simulink model "concept3_simulink_RL"  (R2025a)
settings: Solver=VariableStepAuto  StartTime=0.0  StopTime=Tf  FixedStep=0.001  MaxStep=0.01  MinStep=0.0001  RelTol=1e-3
InitFcn:
  | loaded_data = load('concept3_for_sim.mat');
  | robot = loaded_data.robot;
  | robot.DataFormat = 'column';
values from neighbouring files (symbols this model uses):
  mass = 40    [RL_main.m]    (also in baseline_sim.m)
  obs_vec = opa    [RL_main.m]    (also in baseline_sim.m)
  port = data(n, :)    [RL_main.m]    (also in baseline_sim.m = port_pos_data(n,:))
  port_num = 10    [RL_main.m]    (also in baseline_sim.m)
  port_target = AB2port(port_num)    [RL_main.m]    (also in baseline_sim.m)
  q0arm = rad2deg([-1.283; -1.622; 2.2761853; -1.8021853; 1.112; 1.859; 0.05328])    [RL_main.m]    (also in baseline_sim.m)
  q0b = [1; 0; 0; 0; 0; 0; 0]    [RL_main.m]    (also in baseline_sim.m = [1;0;0;0;0;0;0])
  sat_docked = AB2port(sat_docked_num)    [RL_main.m]    (also in baseline_sim.m)
  sat_docked_num = 6    [RL_main.m]    (also in baseline_sim.m)
  sim_state = 1    [RL_main.m]    (also in baseline_sim.m)
  Tlog = 0.1    [RL_main.m]    (also in baseline_sim.m)
  use_RL = 1    [RL_main.m]    (also in baseline_sim.m)
undefined symbols (not defined in the file or in its folder): opa, target, X, Y, Z
libraries: sm_lib x133, nesl_utility x67, simulink_extras x3, rllib x2
(part 2 of 6)

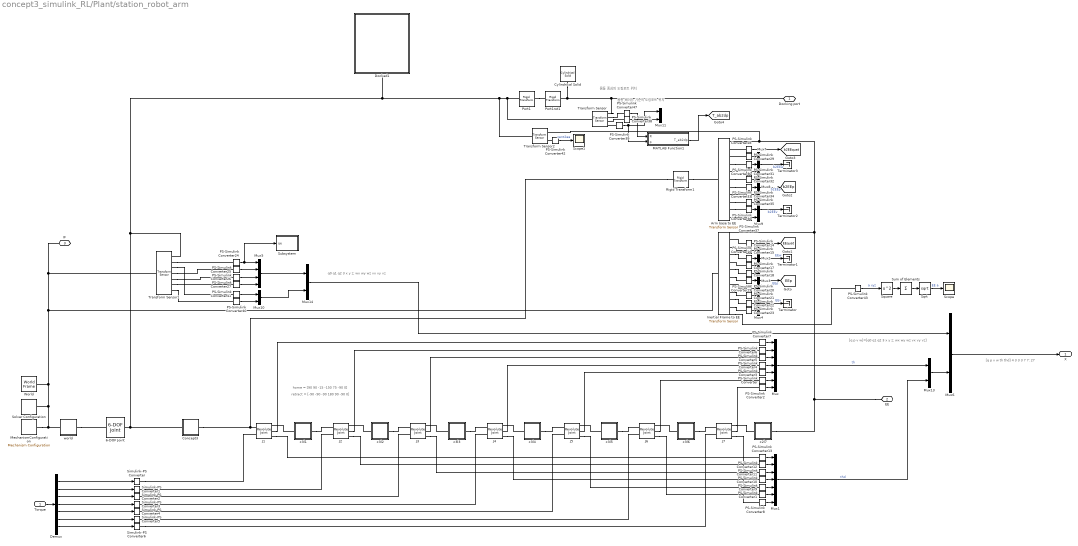
== system concept3_simulink_RL/Plant/station_robot_arm ==
  note: [q p v w th thd]
      |
      | 4 3 3 3 7 7: 27
  note: q0 q1 q2 3 x y z; wx wy wz vx vy vz
  note: 몸통 중심의 도킹포트 위치
  note: home = [90 90 -15 -150 75 -90 0]
  note: retract = [-90 -90 -90 180 90 -90 0]
  note: 몸통 베이스 기준의 도킹포트 위치
  note: [q p v w]=[q0 q1 q2 3 x y z; wx wy wz vx vy vz]
  Torque : Inport
  6-DOF Joint : sm_lib/Joints/6-DOF Joint  JointMode=Normal  CompositeWrenchDir=FollowerOnBase  CompositeWrenchFrame=BaseFrame  SenseConstraintForce=off  SenseConstraintTorque=off  SenseTotalForce=off  SenseTotalTorque=off  PxPositionTargetSpecify=on  PxPositionTargetPriority=High  PxPositionTargetValue=q0b(5)  PxPositionTargetValueUnits=m  PxVelocityTargetSpecify=off  PxVelocityTargetPriority=High  PxVelocityTargetValue=0  PxVelocityTargetValueUnits=m/s  PxEquilibriumPosition=0  PxEquilibriumPositionUnits=m  PxSpringStiffness=0  PxSpringStiffnessUnits=N/m  PxDampingCoefficient=0  PxDampingCoefficientUnits=N/(m/s)  PxLowerLimitSpecify=off  PxLowerLimitBound=-1  PxLowerLimitBoundUnits=m  PxLowerLimitStiffness=1e6  PxLowerLimitStiffnessUnits=N/m  PxLowerLimitDamping=1e3  PxLowerLimitDampingUnits=N/(m/s)  PxLowerLimitTransitionRegionWidth=1e-4  PxLowerLimitTransitionRegionWidthUnits=m  PxUpperLimitSpecify=off  PxUpperLimitBound=1  PxUpperLimitBoundUnits=m  PxUpperLimitStiffness=1e6  PxUpperLimitStiffnessUnits=N/m  PxUpperLimitDamping=1e3  PxUpperLimitDampingUnits=N/(m/s)  PxUpperLimitTransitionRegionWidth=1e-4  PxUpperLimitTransitionRegionWidthUnits=m  PxTorqueActuationMode=NoTorque  PxMotionActuationMode=ComputedMotion  PxSensePosition=off  PxSenseVelocity=off  PxSenseAcceleration=off  PxSenseTorqueForce=off  PxSenseLowerLimitTorqueForce=off  PxSenseUpperLimitTorqueForce=off  PyPositionTargetSpecify=on  PyPositionTargetPriority=High  PyPositionTargetValue=q0b(6)  PyPositionTargetValueUnits=m  PyVelocityTargetSpecify=off  PyVelocityTargetPriority=High  PyVelocityTargetValue=0  PyVelocityTargetValueUnits=m/s  PyEquilibriumPosition=0  PyEquilibriumPositionUnits=m  PySpringStiffness=0  PySpringStiffnessUnits=N/m  PyDampingCoefficient=0  PyDampingCoefficientUnits=N/(m/s)  PyLowerLimitSpecify=off  PyLowerLimitBound=-1  PyLowerLimitBoundUnits=m  PyLowerLimitStiffness=1e6  PyLowerLimitStiffnessUnits=N/m  PyLowerLimitDamping=1e3  PyLowerLimitDampingUnits=N/(m/s)  PyLowerLimitTransitionRegionWidth=1e-4  PyLowerLimitTransitionRegionWidthUnits=m  PyUpperLimitSpecify=off  PyUpperLimitBound=1  PyUpperLimitBoundUnits=m  PyUpperLimitStiffness=1e6  PyUpperLimitStiffnessUnits=N/m  PyUpperLimitDamping=1e3  PyUpperLimitDampingUnits=N/(m/s)  PyUpperLimitTransitionRegionWidth=1e-4  PyUpperLimitTransitionRegionWidthUnits=m  PyTorqueActuationMode=NoTorque  PyMotionActuationMode=ComputedMotion  PySensePosition=off  PySenseVelocity=off  PySenseAcceleration=off  PySenseTorqueForce=off  PySenseLowerLimitTorqueForce=off  PySenseUpperLimitTorqueForce=off  PzPositionTargetSpecify=on  PzPositionTargetPriority=High  PzPositionTargetValue=q0b(7)  PzPositionTargetValueUnits=m  PzVelocityTargetSpecify=off  PzVelocityTargetPriority=High  PzVelocityTargetValue=0  PzVelocityTargetValueUnits=m/s  PzEquilibriumPosition=0  PzEquilibriumPositionUnits=m  PzSpringStiffness=0  PzSpringStiffnessUnits=N/m  PzDampingCoefficient=0  PzDampingCoefficientUnits=N/(m/s)  PzLowerLimitSpecify=off  PzLowerLimitBound=-1  PzLowerLimitBoundUnits=m  PzLowerLimitStiffness=1e6  PzLowerLimitStiffnessUnits=N/m  PzLowerLimitDamping=1e3  PzLowerLimitDampingUnits=N/(m/s)  PzLowerLimitTransitionRegionWidth=1e-4  PzLowerLimitTransitionRegionWidthUnits=m  PzUpperLimitSpecify=off  PzUpperLimitBound=1  PzUpperLimitBoundUnits=m  PzUpperLimitStiffness=1e6  PzUpperLimitStiffnessUnits=N/m  PzUpperLimitDamping=1e3  PzUpperLimitDampingUnits=N/(m/s)  PzUpperLimitTransitionRegionWidth=1e-4  PzUpperLimitTransitionRegionWidthUnits=m  PzTorqueActuationMode=NoTorque  PzMotionActuationMode=ComputedMotion  PzSensePosition=off  PzSenseVelocity=off  PzSenseAcceleration=off  PzSenseTorqueForce=off  PzSenseLowerLimitTorqueForce=off  PzSenseUpperLimitTorqueForce=off  SphPositionTargetSpecify=on  SphPositionTargetPriority=High  SphPositionTargetRotationMethod=Quaternion  SphPositionTargetFollAlignAxisA=+X  SphPositionTargetBaseAlignAxisA=+Y  SphPositionTargetFollAlignAxisB=+Y  SphPositionTargetBaseAlignAxisB=+Z  SphPositionTargetRotationStandardAxis=+Y  SphPositionTargetRotationAngle=0  SphPositionTargetRotationAngleUnits=deg  SphPositionTargetRotationArbitraryAxis=[0 0 1]  SphPositionTargetRotationSequenceAxes=FollowerAxes  SphPositionTargetRotationSequence=XYX  SphPositionTargetRotationSequenceAngles=[0 0 0]  SphPositionTargetRotationSequenceAnglesUnits=deg  SphPositionTargetRotationMatrix=[1 0 0;0 1 0;0 0 1]  SphPositionTargetQuaternion=q0b(1:4)  SphVelocityTargetSpecify=off  SphVelocityTargetPriority=High  SphVelocityTargetValue=[0 0 0]  SphVelocityTargetValueUnits=deg/s  SphVelocityTargetInFollowerFrame=on  SphEqPosRotationMethod=None  SphEqPosFollAlignAxisA=+X  SphEqPosBaseAlignAxisA=+Y  SphEqPosFollAlignAxisB=+Y  SphEqPosBaseAlignAxisB=+Z  SphEqPosRotationStandardAxis=+Z  SphEqPosRotationAngle=0  SphEqPosRotationAngleUnits=deg  SphEqPosRotationArbitraryAxis=[0 0 1]  SphEqPosRotationSequenceAxes=FollowerAxes  SphEqPosRotationSequence=XYX  SphEqPosRotationSequenceAngles=[0 0 0]  SphEqPosRotationSequenceAnglesUnits=deg  SphEqPosRotationMatrix=[1 0 0;0 1 0;0 0 1]  SphEqPosQuaternion=[1 0 0 0]  SphSpringStiffness=0  SphSpringStiffnessUnits=N*m/deg  SphDampingCoefficient=0  SphDampingCoefficientUnits=N*m/(deg/s)  SphLowerLimitSpecify=off  SphLowerLimitBound=15  SphLowerLimitBoundUnits=deg  SphLowerLimitStiffness=1e4  SphLowerLimitStiffnessUnits=N*m/deg  SphLowerLimitDamping=10  SphLowerLimitDampingUnits=N*m/(deg/s)  SphLowerLimitTransitionRegionWidth=0.1  SphLowerLimitTransitionRegionWidthUnits=deg  SphUpperLimitSpecify=off  SphUpperLimitBound=45  SphUpperLimitBoundUnits=deg  SphUpperLimitStiffness=1e4  SphUpperLimitStiffnessUnits=N*m/deg  SphUpperLimitDamping=10  SphUpperLimitDampingUnits=N*m/(deg/s)  SphUpperLimitTransitionRegionWidth=0.1  SphUpperLimitTransitionRegionWidthUnits=deg  SphTorqueActuationMode=InputTorque  SphActuateTorqueX=off  SphActuateTorqueY=off  SphActuateTorqueZ=off  SphActuateTorque=off  SphActuationFrame=BaseFrame  SphSensePosition=off  SphSenseVelocityX=off  SphSenseVelocityY=off  SphSenseVelocityZ=off  SphSenseVelocity=off  SphSenseAccelerationX=off  SphSenseAccelerationY=off  SphSenseAccelerationZ=off  SphSenseAcceleration=off  SphSenseLowerLimitTorqueMag=off  SphSenseUpperLimitTorqueMag=off  SphSensingFrame=BaseFrame
  Arm base to EE : sm_lib/Frames and Transforms/Transform Sensor  MeasurementFrame=Base  RotationSequence=XYX  SenseAngle=off  SenseAxis=off  SenseQ=on  SenseR=off  SenseRotationSequence=off  SenseOmegaX=on  SenseOmegaY=on  SenseOmegaZ=on  SenseOmega=off  SenseQDot=off  SenseRDot=off  SenseRotationSequenceDot=off  SenseAlphaX=off  SenseAlphaY=off  SenseAlphaZ=off  SenseAlpha=off  SenseQDDot=off  SenseRDDot=off  SenseX=on  SenseY=on  SenseZ=on  SenseXYZ=off  SenseRad=off  SenseAzim=off  SenseDist=off  SenseInc=off  SenseXDot=on  SenseYDot=on  SenseZDot=on  SenseXYZDot=off  SenseRadDot=off  SenseAzimDot=off  SenseDistDot=off  SenseIncDot=off  SenseXDDot=off  SenseYDDot=off  SenseZDDot=off  SenseXYZDDot=off  SenseRadDDot=off  SenseAzimDDot=off  SenseDistDDot=off  SenseIncDDot=off
  Concept3 : Subsystem
  Cylindrical Solid : sm_lib/Body Elements/Cylindrical Solid  CylinderRadius=0.05  CylinderRadiusUnits=m  CylinderLength=0.01  CylinderLengthUnits=m  ExportEntireGeometry=off  InertiaType=CalculateFromGeometry  BasedOnType=Mass  Density=1000  DensityUnits=kg/m^3  Mass=0  MassUnits=kg  CenterOfMass=[0 0 0]  CenterOfMassUnits=m  MomentsOfInertia=[1 1 1]  MomentsOfInertiaUnits=kg*m^2  ProductsOfInertia=[0 0 0]  ProductsOfInertiaUnits=kg*m^2  GraphicType=FromGeometry  MarkerShape=Sphere  MarkerSize=10  GraphicVisPropType=SimpleVisualProperties  GraphicDiffuseColor=[0 1 1]  GraphicOpacity=0.5  GraphicSpecularColor=[0.5 0.5 0.5 1]  GraphicAmbientColor=[0.15 0.15 0.15 1]  GraphicEmissiveColor=[0.0 0.0 0.0 1.0]  GraphicShininess=100  DoExposeReferenceFrame=on  SerializedFrames=<Frames/>
  Demux : Demux  Outputs=7
  Docked1 : Subsystem
  Inertial Frame to EE : sm_lib/Frames and Transforms/Transform Sensor  MeasurementFrame=World  RotationSequence=XYX  SenseAngle=off  SenseAxis=off  SenseQ=on  SenseR=off  SenseRotationSequence=off  SenseOmegaX=on  SenseOmegaY=on  SenseOmegaZ=on  SenseOmega=off  SenseQDot=off  SenseRDot=off  SenseRotationSequenceDot=off  SenseAlphaX=off  SenseAlphaY=off  SenseAlphaZ=off  SenseAlpha=off  SenseQDDot=off  SenseRDDot=off  SenseX=on  SenseY=on  SenseZ=on  SenseXYZ=off  SenseRad=off  SenseAzim=off  SenseDist=off  SenseInc=off  SenseXDot=on  SenseYDot=on  SenseZDot=on  SenseXYZDot=off  SenseRadDot=off  SenseAzimDot=off  SenseDistDot=off  SenseIncDot=off  SenseXDDot=off  SenseYDDot=off  SenseZDDot=off  SenseXYZDDot=on  SenseRadDDot=off  SenseAzimDDot=off  SenseDistDDot=off  SenseIncDDot=off
  J1 : sm_lib/Joints/Revolute Joint  JointMode=Normal  CompositeWrenchDir=FollowerOnBase  CompositeWrenchFrame=BaseFrame  SenseConstraintForce=off  SenseConstraintTorque=off  SenseTotalForce=off  SenseTotalTorque=off  PositionTargetSpecify=on  PositionTargetPriority=High  PositionTargetValue=q0arm(1)  PositionTargetValueUnits=deg  VelocityTargetSpecify=off  VelocityTargetPriority=High  VelocityTargetValue=0  VelocityTargetValueUnits=deg/s  EquilibriumPosition=0  EquilibriumPositionUnits=deg  SpringStiffness=0  SpringStiffnessUnits=N*m/deg  DampingCoefficient=0  DampingCoefficientUnits=kg*m^2/(rad*s)  LowerLimitSpecify=off  LowerLimitBound=-90  LowerLimitBoundUnits=deg  LowerLimitStiffness=1e4  LowerLimitStiffnessUnits=N*m/deg  LowerLimitDamping=10  LowerLimitDampingUnits=N*m/(deg/s)  LowerLimitTransitionRegionWidth=0.1  LowerLimitTransitionRegionWidthUnits=deg  UpperLimitSpecify=off  UpperLimitBound=90  UpperLimitBoundUnits=deg  UpperLimitStiffness=1e4  UpperLimitStiffnessUnits=N*m/deg  UpperLimitDamping=10  UpperLimitDampingUnits=N*m/(deg/s)  UpperLimitTransitionRegionWidth=0.1  UpperLimitTransitionRegionWidthUnits=deg  TorqueActuationMode=InputTorque  MotionActuationMode=ComputedMotion  SensePosition=on  SenseVelocity=on  SenseAcceleration=off  SenseTorqueForce=off  SenseLowerLimitTorqueForce=off  SenseUpperLimitTorqueForce=off
  J2 : sm_lib/Joints/Revolute Joint  JointMode=Normal  CompositeWrenchDir=FollowerOnBase  CompositeWrenchFrame=BaseFrame  SenseConstraintForce=off  SenseConstraintTorque=off  SenseTotalForce=off  SenseTotalTorque=off  PositionTargetSpecify=on  PositionTargetPriority=High  PositionTargetValue=q0arm(2)  PositionTargetValueUnits=deg  VelocityTargetSpecify=off  VelocityTargetPriority=High  VelocityTargetValue=0  VelocityTargetValueUnits=deg/s  EquilibriumPosition=0  EquilibriumPositionUnits=deg  SpringStiffness=0  SpringStiffnessUnits=N*m/deg  DampingCoefficient=0  DampingCoefficientUnits=kg*m^2/(rad*s)  LowerLimitSpecify=off  LowerLimitBound=-90  LowerLimitBoundUnits=deg  LowerLimitStiffness=1e4  LowerLimitStiffnessUnits=N*m/deg  LowerLimitDamping=10  LowerLimitDampingUnits=N*m/(deg/s)  LowerLimitTransitionRegionWidth=0.1  LowerLimitTransitionRegionWidthUnits=deg  UpperLimitSpecify=off  UpperLimitBound=90  UpperLimitBoundUnits=deg  UpperLimitStiffness=1e4  UpperLimitStiffnessUnits=N*m/deg  UpperLimitDamping=10  UpperLimitDampingUnits=N*m/(deg/s)  UpperLimitTransitionRegionWidth=0.1  UpperLimitTransitionRegionWidthUnits=deg  TorqueActuationMode=InputTorque  MotionActuationMode=ComputedMotion  SensePosition=on  SenseVelocity=on  SenseAcceleration=off  SenseTorqueForce=off  SenseLowerLimitTorqueForce=off  SenseUpperLimitTorqueForce=off
  J3 : sm_lib/Joints/Revolute Joint  JointMode=Normal  CompositeWrenchDir=FollowerOnBase  CompositeWrenchFrame=BaseFrame  SenseConstraintForce=off  SenseConstraintTorque=off  SenseTotalForce=off  SenseTotalTorque=off  PositionTargetSpecify=on  PositionTargetPriority=High  PositionTargetValue=q0arm(3)  PositionTargetValueUnits=deg  VelocityTargetSpecify=off  VelocityTargetPriority=High  VelocityTargetValue=0  VelocityTargetValueUnits=deg/s  EquilibriumPosition=0  EquilibriumPositionUnits=deg  SpringStiffness=0  SpringStiffnessUnits=N*m/deg  DampingCoefficient=0  DampingCoefficientUnits=kg*m^2/(rad*s)  LowerLimitSpecify=off  LowerLimitBound=-90  LowerLimitBoundUnits=deg  LowerLimitStiffness=1e4  LowerLimitStiffnessUnits=N*m/deg  LowerLimitDamping=10  LowerLimitDampingUnits=N*m/(deg/s)  LowerLimitTransitionRegionWidth=0.1  LowerLimitTransitionRegionWidthUnits=deg  UpperLimitSpecify=off  UpperLimitBound=90  UpperLimitBoundUnits=deg  UpperLimitStiffness=1e4  UpperLimitStiffnessUnits=N*m/deg  UpperLimitDamping=10  UpperLimitDampingUnits=N*m/(deg/s)  UpperLimitTransitionRegionWidth=0.1  UpperLimitTransitionRegionWidthUnits=deg  TorqueActuationMode=InputTorque  MotionActuationMode=ComputedMotion  SensePosition=on  SenseVelocity=on  SenseAcceleration=off  SenseTorqueForce=off  SenseLowerLimitTorqueForce=off  SenseUpperLimitTorqueForce=off
  J4 : sm_lib/Joints/Revolute Joint  JointMode=Normal  CompositeWrenchDir=FollowerOnBase  CompositeWrenchFrame=BaseFrame  SenseConstraintForce=off  SenseConstraintTorque=off  SenseTotalForce=off  SenseTotalTorque=off  PositionTargetSpecify=on  PositionTargetPriority=High  PositionTargetValue=q0arm(4)  PositionTargetValueUnits=deg  VelocityTargetSpecify=off  VelocityTargetPriority=High  VelocityTargetValue=0  VelocityTargetValueUnits=deg/s  EquilibriumPosition=0  EquilibriumPositionUnits=deg  SpringStiffness=0  SpringStiffnessUnits=N*m/deg  DampingCoefficient=0  DampingCoefficientUnits=kg*m^2/(rad*s)  LowerLimitSpecify=off  LowerLimitBound=-90  LowerLimitBoundUnits=deg  LowerLimitStiffness=1e4  LowerLimitStiffnessUnits=N*m/deg  LowerLimitDamping=10  LowerLimitDampingUnits=N*m/(deg/s)  LowerLimitTransitionRegionWidth=0.1  LowerLimitTransitionRegionWidthUnits=deg  UpperLimitSpecify=off  UpperLimitBound=90  UpperLimitBoundUnits=deg  UpperLimitStiffness=1e4  UpperLimitStiffnessUnits=N*m/deg  UpperLimitDamping=10  UpperLimitDampingUnits=N*m/(deg/s)  UpperLimitTransitionRegionWidth=0.1  UpperLimitTransitionRegionWidthUnits=deg  TorqueActuationMode=InputTorque  MotionActuationMode=ComputedMotion  SensePosition=on  SenseVelocity=on  SenseAcceleration=off  SenseTorqueForce=off  SenseLowerLimitTorqueForce=off  SenseUpperLimitTorqueForce=off
  J5 : sm_lib/Joints/Revolute Joint  JointMode=Normal  CompositeWrenchDir=FollowerOnBase  CompositeWrenchFrame=BaseFrame  SenseConstraintForce=off  SenseConstraintTorque=off  SenseTotalForce=off  SenseTotalTorque=off  PositionTargetSpecify=on  PositionTargetPriority=High  PositionTargetValue=q0arm(5)  PositionTargetValueUnits=deg  VelocityTargetSpecify=off  VelocityTargetPriority=High  VelocityTargetValue=0  VelocityTargetValueUnits=deg/s  EquilibriumPosition=0  EquilibriumPositionUnits=deg  SpringStiffness=0  SpringStiffnessUnits=N*m/deg  DampingCoefficient=0  DampingCoefficientUnits=kg*m^2/(rad*s)  LowerLimitSpecify=off  LowerLimitBound=-90  LowerLimitBoundUnits=deg  LowerLimitStiffness=1e4  LowerLimitStiffnessUnits=N*m/deg  LowerLimitDamping=10  LowerLimitDampingUnits=N*m/(deg/s)  LowerLimitTransitionRegionWidth=0.1  LowerLimitTransitionRegionWidthUnits=deg  UpperLimitSpecify=off  UpperLimitBound=90  UpperLimitBoundUnits=deg  UpperLimitStiffness=1e4  UpperLimitStiffnessUnits=N*m/deg  UpperLimitDamping=10  UpperLimitDampingUnits=N*m/(deg/s)  UpperLimitTransitionRegionWidth=0.1  UpperLimitTransitionRegionWidthUnits=deg  TorqueActuationMode=InputTorque  MotionActuationMode=ComputedMotion  SensePosition=on  SenseVelocity=on  SenseAcceleration=off  SenseTorqueForce=off  SenseLowerLimitTorqueForce=off  SenseUpperLimitTorqueForce=off
  J6 : sm_lib/Joints/Revolute Joint  JointMode=Normal  CompositeWrenchDir=FollowerOnBase  CompositeWrenchFrame=BaseFrame  SenseConstraintForce=off  SenseConstraintTorque=off  SenseTotalForce=off  SenseTotalTorque=off  PositionTargetSpecify=on  PositionTargetPriority=High  PositionTargetValue=q0arm(6)  PositionTargetValueUnits=deg  VelocityTargetSpecify=off  VelocityTargetPriority=High  VelocityTargetValue=0  VelocityTargetValueUnits=deg/s  EquilibriumPosition=0  EquilibriumPositionUnits=deg  SpringStiffness=0  SpringStiffnessUnits=N*m/deg  DampingCoefficient=0  DampingCoefficientUnits=kg*m^2/(rad*s)  LowerLimitSpecify=off  LowerLimitBound=-90  LowerLimitBoundUnits=deg  LowerLimitStiffness=1e4  LowerLimitStiffnessUnits=N*m/deg  LowerLimitDamping=10  LowerLimitDampingUnits=N*m/(deg/s)  LowerLimitTransitionRegionWidth=0.1  LowerLimitTransitionRegionWidthUnits=deg  UpperLimitSpecify=off  UpperLimitBound=90  UpperLimitBoundUnits=deg  UpperLimitStiffness=1e4  UpperLimitStiffnessUnits=N*m/deg  UpperLimitDamping=10  UpperLimitDampingUnits=N*m/(deg/s)  UpperLimitTransitionRegionWidth=0.1  UpperLimitTransitionRegionWidthUnits=deg  TorqueActuationMode=InputTorque  MotionActuationMode=ComputedMotion  SensePosition=on  SenseVelocity=on  SenseAcceleration=off  SenseTorqueForce=off  SenseLowerLimitTorqueForce=off  SenseUpperLimitTorqueForce=off
  J7 : sm_lib/Joints/Revolute Joint  JointMode=Normal  CompositeWrenchDir=FollowerOnBase  CompositeWrenchFrame=BaseFrame  SenseConstraintForce=off  SenseConstraintTorque=off  SenseTotalForce=off  SenseTotalTorque=off  PositionTargetSpecify=on  PositionTargetPriority=High  PositionTargetValue=q0arm(7)  PositionTargetValueUnits=deg  VelocityTargetSpecify=off  VelocityTargetPriority=High  VelocityTargetValue=0  VelocityTargetValueUnits=deg/s  EquilibriumPosition=0  EquilibriumPositionUnits=deg  SpringStiffness=0  SpringStiffnessUnits=N*m/deg  DampingCoefficient=0  DampingCoefficientUnits=kg*m^2/(rad*s)  LowerLimitSpecify=off  LowerLimitBound=-90  LowerLimitBoundUnits=deg  LowerLimitStiffness=1e4  LowerLimitStiffnessUnits=N*m/deg  LowerLimitDamping=10  LowerLimitDampingUnits=N*m/(deg/s)  LowerLimitTransitionRegionWidth=0.1  LowerLimitTransitionRegionWidthUnits=deg  UpperLimitSpecify=off  UpperLimitBound=90  UpperLimitBoundUnits=deg  UpperLimitStiffness=1e4  UpperLimitStiffnessUnits=N*m/deg  UpperLimitDamping=10  UpperLimitDampingUnits=N*m/(deg/s)  UpperLimitTransitionRegionWidth=0.1  UpperLimitTransitionRegionWidthUnits=deg  TorqueActuationMode=InputTorque  MotionActuationMode=ComputedMotion  SensePosition=on  SenseVelocity=on  SenseAcceleration=off  SenseTorqueForce=off  SenseLowerLimitTorqueForce=off  SenseUpperLimitTorqueForce=off
  MATLAB Function1 : MATLAB Function  TreatAsAtomicUnit=on
  MechanismConfiguration : sm_lib/Utilities/Mechanism Configuration  UniformGravity=Constant  GravityVector=[0, 0, 0]  GravityVectorUnits=m/s^2  LinearizationDelta=0.001  JointModeTransitionNonlinearIterations=2
  Mux : Mux  Inputs=7
  Mux1 : Mux  Inputs=7
  Mux{6,10..11,13..14} (5 alike) : Mux  Inputs=2
  Mux{2..4,7..9} (6 alike) : Mux  Inputs=3
  Mux5 : Mux
  PS-Simulink Converter{,1..43,47} (45 alike) : nesl_utility/PS-Simulink Converter  PhysicalDomain=network_engine_domain  SubClassName=ps_output  LeftPortType=input  RightPortType=output  PseudoPeriodic=off  Frequencies=[]  VectorFormat=inherit  Unit=inherit  AffineConversion=off
  Port1 : sm_lib/Frames and Transforms/Rigid Transform  RotationMethod=None  FollAlignAxisA=+X  BaseAlignAxisA=+Y  FollAlignAxisB=+Y  BaseAlignAxisB=+Z  RotationStandardAxis=+Z  RotationAngle=0  RotationAngleUnits=deg  RotationArbitraryAxis=[0 0 1]  RotationSequenceAxes=FollowerAxes  RotationSequence=XYX  RotationSequenceAngles=[0 0 0]  RotationSequenceAnglesUnits=deg  RotationMatrix=[1 0 0;0 1 0;0 0 1]  Quaternion=[1 0 0 0]  TranslationMethod=Cartesian  TranslationCartesianOffset=port_target(1:3)  TranslationCartesianOffsetUnits=m  TranslationStandardAxis=+Z  TranslationStandardOffset=0  TranslationStandardOffsetUnits=m  TranslationROffset=0  TranslationROffsetUnits=m  TranslationThetaOffset=0  TranslationThetaOffsetUnits=deg  TranslationZOffset=0  TranslationZOffsetUnits=m
  Port1rot1 : sm_lib/Frames and Transforms/Rigid Transform  RotationMethod=RotationSequence  FollAlignAxisA=+X  BaseAlignAxisA=+Y  FollAlignAxisB=+Y  BaseAlignAxisB=+Z  RotationStandardAxis=+Z  RotationAngle=0  RotationAngleUnits=deg  RotationArbitraryAxis=[0 0 1]  RotationSequenceAxes=FollowerAxes  RotationSequence=ZYX  RotationSequenceAngles=port_target(4:6)  RotationSequenceAnglesUnits=deg  RotationMatrix=[1 0 0;0 1 0;0 0 1]  Quaternion=[1 0 0 0]  TranslationMethod=None  TranslationCartesianOffset=[0.9 -0.25 -0.05]  TranslationCartesianOffsetUnits=m  TranslationStandardAxis=+Z  TranslationStandardOffset=0  TranslationStandardOffsetUnits=m  TranslationROffset=0  TranslationROffsetUnits=m  TranslationThetaOffset=0  TranslationThetaOffsetUnits=deg  TranslationZOffset=0  TranslationZOffsetUnits=m
  Rigid Transform1 : sm_lib/Frames and Transforms/Rigid Transform  RotationMethod=StandardAxis  FollAlignAxisA=+X  BaseAlignAxisA=+Y  FollAlignAxisB=+Y  BaseAlignAxisB=+Z  RotationStandardAxis=+Z  RotationAngle=0  RotationAngleUnits=deg  RotationArbitraryAxis=[0 0 1]  RotationSequenceAxes=FollowerAxes  RotationSequence=XYX  RotationSequenceAngles=[0 0 0]  RotationSequenceAnglesUnits=deg  RotationMatrix=[1 0 0;0 1 0;0 0 1]  Quaternion=[1 0 0 0]  TranslationMethod=None  TranslationCartesianOffset=[0 0 0]  TranslationCartesianOffsetUnits=m  TranslationStandardAxis=+Z  TranslationStandardOffset=0  TranslationStandardOffsetUnits=m  TranslationROffset=0  TranslationROffsetUnits=m  TranslationThetaOffset=0  TranslationThetaOffsetUnits=deg  TranslationZOffset=0  TranslationZOffsetUnits=m
  Scope : Scope
  Scope1 : Scope
      settings: DataLoggingVariableName=ScopeData3
  Simulink-PS Converter{,1..6} (7 alike) : nesl_utility/Simulink-PS Converter  PhysicalDomain=network_engine_domain  SubClassName=ps_input  LeftPortType=input  RightPortType=output  PseudoPeriodic=off  Frequencies=[]  NoiseDistribution=none  NoiseParameters=[]  Unit=1  AffineConversion=off  FilteringAndDerivatives=provide  SimscapeFilterOrder=1  InputFilterTimeConstant=0.001  UdotUserProvided=0
  Solver Configuration : nesl_utility/Solver Configuration  PhysicalDomain=network_engine_domain  SubClassName=solver  LeftPortType=input  RightPortType=generic  Tones=[]  Harmonics=[]  SimulateNoise=off  Profile=off  UseLocalSampling=off  EnableSwitchedLinearOptims=on  FrequencyDomain=off  UseCCode=off  RelTol=0.001  AbsTol=0.001  MinStep=1e-09  ToWorkspace=off  RevertToSquareIcSolve=off  NumHomotopyIterations=100  PhasorMode=off  PhasorModeNumHarmonics=1  ConsistencySolver=NEWTON_XTOL_AFTER_FTOL  IndexReductionMethod=DerivativeReplacement  DoDC=off  ResidualTolerance=1e-09  ConsistencyTolSource=GLOBAL  ConsistencyAbsTol=0.001  ConsistencyRelTol=0.001  ConsistencyTolFactor=0.001  UseLocalSolver=off  LocalSolverChoice=NE_BACKWARD_EULER_ADVANCER  ResolveIndetEquations=on  FunctionEvalNumThread=1  LocalSolverSampleTime=0.001  DoFixedCost=off  MaxNonlinIter=3  MaxModeIter=2  ComputeImpulses=off  ImpulseIterations=2  LinearAlgebra=auto  LinearAlgebraNumThread=0  EquationFormulation=NE_TIME_EF  DelaysMemoryBudget=1024  AutomaticFiltering=on  FilteringTimeConstant=0.001  PartitionStorageMethod=AS_NEEDED  PartitionMemoryBudget=1024  PartitionMethod=ROBUST  MultibodyUseLocalSolver=off  MultibodyLocalSolverChoice=ODE1  MultibodyLocalSolverSampleTime=0.001
  Sqrt : Sqrt
  Square : Math  Operator=square
  Subsystem : Subsystem
  Sum of Elements : Sum  Inputs=+
  Terminator{,1..3} (4 alike) : Terminator
  Transform Sensor : sm_lib/Frames and Transforms/Transform Sensor  MeasurementFrame=Base  RotationSequence=ZYX  SenseAngle=off  SenseAxis=off  SenseQ=off  SenseR=on  SenseRotationSequence=on  SenseOmegaX=off  SenseOmegaY=off  SenseOmegaZ=off  SenseOmega=off  SenseQDot=off  SenseRDot=off  SenseRotationSequenceDot=off  SenseAlphaX=off  SenseAlphaY=off  SenseAlphaZ=off  SenseAlpha=off  SenseQDDot=off  SenseRDDot=off  SenseX=off  SenseY=off  SenseZ=off  SenseXYZ=on  SenseRad=off  SenseAzim=off  SenseDist=off  SenseInc=off  SenseXDot=off  SenseYDot=off  SenseZDot=off  SenseXYZDot=off  SenseRadDot=off  SenseAzimDot=off  SenseDistDot=off  SenseIncDot=off  SenseXDDot=off  SenseYDDot=off  SenseZDDot=off  SenseXYZDDot=off  SenseRadDDot=off  SenseAzimDDot=off  SenseDistDDot=off  SenseIncDDot=off
  Transform Sensor1 : sm_lib/Frames and Transforms/Transform Sensor  MeasurementFrame=World  RotationSequence=XYX  SenseAngle=off  SenseAxis=off  SenseQ=on  SenseR=off  SenseRotationSequence=off  SenseOmegaX=off  SenseOmegaY=off  SenseOmegaZ=off  SenseOmega=on  SenseQDot=off  SenseRDot=off  SenseRotationSequenceDot=off  SenseAlphaX=off  SenseAlphaY=off  SenseAlphaZ=off  SenseAlpha=off  SenseQDDot=off  SenseRDDot=off  SenseX=on  SenseY=on  SenseZ=on  SenseXYZ=off  SenseRad=off  SenseAzim=off  SenseDist=off  SenseInc=off  SenseXDot=off  SenseYDot=off  SenseZDot=off  SenseXYZDot=on  SenseRadDot=off  SenseAzimDot=off  SenseDistDot=off  SenseIncDot=off  SenseXDDot=off  SenseYDDot=off  SenseZDDot=off  SenseXYZDDot=off  SenseRadDDot=off  SenseAzimDDot=off  SenseDistDDot=off  SenseIncDDot=off
  Transform Sensor2 : sm_lib/Frames and Transforms/Transform Sensor  MeasurementFrame=Base  RotationSequence=ZYX  SenseAngle=off  SenseAxis=off  SenseQ=off  SenseR=off  SenseRotationSequence=off  SenseOmegaX=off  SenseOmegaY=off  SenseOmegaZ=off  SenseOmega=off  SenseQDot=off  SenseRDot=off  SenseRotationSequenceDot=off  SenseAlphaX=off  SenseAlphaY=off  SenseAlphaZ=off  SenseAlpha=off  SenseQDDot=off  SenseRDDot=off  SenseX=off  SenseY=off  SenseZ=off  SenseXYZ=on  SenseRad=off  SenseAzim=off  SenseDist=off  SenseInc=off  SenseXDot=off  SenseYDot=off  SenseZDot=off  SenseXYZDot=off  SenseRadDot=off  SenseAzimDot=off  SenseDistDot=off  SenseIncDot=off  SenseXDDot=off  SenseYDDot=off  SenseZDDot=off  SenseXYZDDot=off  SenseRadDDot=off  SenseAzimDDot=off  SenseDistDDot=off  SenseIncDDot=off
  World : sm_lib/Frames and Transforms/World Frame
  c2l7 : Subsystem
  c3l1 : Subsystem
  c3l2 : Subsystem
  c3l3 : Subsystem
  c3l4 : Subsystem
  c3l5 : Subsystem
  c3l6 : Subsystem
  world : Subsystem
  Docking port : PMIOPort  Side=Right
  EE : PMIOPort  Port=2  Side=Right
  IF : PMIOPort  Port=3  Side=Right
  X : Outport
  tag scope: EEp=global, EEquat=global, T_ab2dp=global, b2EEp=global, b2EEquat=global
  wires:
  PS-Simulink Converter4/1 -> Mux/4
  Mux4/1 -> Terminator/1  "EEv"
  Demux/5 -> Simulink-PS Converter4/1
  PS-Simulink Converter9/1 -> Mux1/5
  PS-Simulink Converter15/1 -> Mux2/1
  Torque/1 -> Demux/1
  PS-Simulink Converter26/1 -> Mux5/3
  PS-Simulink Converter13/1 -> Mux1/1
  PS-Simulink Converter8/1 -> Mux1/7
  Mux2/1 -> Terminator1/1  "EEw"
  PS-Simulink Converter23/1 -> Mux4/3
  PS-Simulink Converter11/1 -> Mux1/3
  PS-Simulink Converter5/1 -> Mux/3
  Demux/4 -> Simulink-PS Converter3/1
  PS-Simulink Converter1/1 -> Mux1/6
  Demux/2 -> Simulink-PS Converter1/1
  PS-Simulink Converter22/1 -> Mux4/2
  PS-Simulink Converter21/1 -> Mux4/1
  Demux/3 -> Simulink-PS Converter2/1
  PS-Simulink Converter19/1 -> Mux3/2
  PS-Simulink Converter6/1 -> Mux/2
  PS-Simulink Converter20/1 -> Mux3/3
  PS-Simulink Converter3/1 -> Mux/5
  PS-Simulink Converter17/1 -> Mux2/3
  PS-Simulink Converter2/1 -> Mux/7
  PS-Simulink Converter16/1 -> Mux2/2
  Demux/1 -> Simulink-PS Converter/1
  PS-Simulink Converter12/1 -> Mux1/2
  Demux/6 -> Simulink-PS Converter5/1
  PS-Simulink Converter25/1 -> Mux5/2
  Mux3/1 -> [EEp]  "EEp"
  PS-Simulink Converter7/1 -> Mux/1
  PS-Simulink Converter27/1 -> Mux5/4
  PS-Simulink Converter14/1 -> [EEquat]
  PS-Simulink Converter/1 -> Mux/6
  PS-Simulink Converter10/1 -> Mux1/4
  PS-Simulink Converter18/1 -> Mux3/1
  PS-Simulink Converter31/1 -> Mux7/3
  PS-Simulink Converter30/1 -> Mux7/2
  PS-Simulink Converter29/1 -> Mux7/1
  Mux7/1 -> Terminator3/1  "b2EEw"
  PS-Simulink Converter34/1 -> Mux8/3
  Mux9/1 -> Terminator2/1  "b2EEv"
  PS-Simulink Converter33/1 -> Mux8/2
  PS-Simulink Converter28/1 -> [b2EEquat]
  PS-Simulink Converter36/1 -> Mux9/2
  PS-Simulink Converter37/1 -> Mux9/3
  PS-Simulink Converter35/1 -> Mux9/1
  Mux8/1 -> [b2EEp]  "b2EEp"
  PS-Simulink Converter32/1 -> Mux8/1
  PS-Simulink Converter38/1 -> Mux11/2
  PS-Simulink Converter39/1 -> MATLAB Function1/2(p), Mux11/1
  PS-Simulink Converter40/1 -> Mux10/2
  PS-Simulink Converter41/1 -> Mux10/1
  PS-Simulink Converter42/1 -> Scope1/1  "cent2ee"
  Demux/7 -> Simulink-PS Converter6/1
  PS-Simulink Converter47/1 -> MATLAB Function1/1(R)
  PS-Simulink Converter43/1 -> Square/1  "a xyz"
  Square/1 -> Sum of Elements/1
  Sum of Elements/1 -> Sqrt/1
  Sqrt/1 -> Scope/1  "EE a"
  MATLAB Function1/1(T_ab2dp) -> [T_ab2dp]
  Mux6/1 -> X/1
  Mux/1 -> Mux13/1  "th"
  Mux1/1 -> Mux13/2  "thd"
  Mux13/1 -> Mux6/2
  Mux5/1 -> Mux14/1
  Mux10/1 -> Mux14/2
  Mux14/1 -> Mux6/1
  PS-Simulink Converter24/1 -> Subsystem/1(qe), Mux5/1
  connections:
  c3l6/RConn1 -- J7/LConn1
  Inertial Frame to EE/RConn9 -- PS-Simulink Converter21/LConn1
  c3l2/RConn1 -- J3/LConn1
  EE/RConn1 -- c2l7/RConn1 -- Inertial Frame to EE/RConn1 -- Transform Sensor2/RConn1 -- Arm base to EE/RConn1
  c3l6/LConn1 -- J6/RConn1
  J1/RConn3 -- PS-Simulink Converter13/LConn1
  PS-Simulink Converter20/LConn1 -- Inertial Frame to EE/RConn8
  MechanismConfiguration/RConn1 -- World/RConn1 -- IF/RConn1 -- Transform Sensor1/LConn1 -- Inertial Frame to EE/LConn1 -- Solver Configuration/RConn1 -- world/LConn1
  Transform Sensor1/RConn4 -- PS-Simulink Converter25/LConn1
  Inertial Frame to EE/RConn10 -- PS-Simulink Converter22/LConn1
  Simulink-PS Converter5/RConn1 -- J6/LConn2
  J5/RConn3 -- PS-Simulink Converter9/LConn1
  PS-Simulink Converter15/LConn1 -- Inertial Frame to EE/RConn3
  c3l3/RConn1 -- J4/LConn1
  Transform Sensor1/RConn2 -- PS-Simulink Converter24/LConn1
  Inertial Frame to EE/RConn7 -- PS-Simulink Converter19/LConn1
  Simulink-PS Converter/RConn1 -- J1/LConn2
  J4/RConn2 -- PS-Simulink Converter4/LConn1
  J2/RConn3 -- PS-Simulink Converter12/LConn1
  c3l5/LConn1 -- J5/RConn1
  J6/RConn2 -- PS-Simulink Converter/LConn1
  Simulink-PS Converter3/RConn1 -- J4/LConn2
  PS-Simulink Converter14/LConn1 -- Inertial Frame to EE/RConn2
  c3l5/RConn1 -- J6/LConn1
  c3l2/LConn1 -- J2/RConn1
  J3/RConn2 -- PS-Simulink Converter5/LConn1
  Transform Sensor1/RConn6 -- PS-Simulink Converter27/LConn1
  PS-Simulink Converter17/LConn1 -- Inertial Frame to EE/RConn5
  Rigid Transform1/LConn1 -- Concept3/RConn1 -- J1/LConn1
  c3l4/LConn1 -- J4/RConn1
  c3l4/RConn1 -- J5/LConn1
  J7/RConn1 -- c2l7/LConn1
  Simulink-PS Converter1/RConn1 -- J2/LConn2
  Inertial Frame to EE/RConn11 -- PS-Simulink Converter23/LConn1
  Simulink-PS Converter2/RConn1 -- J3/LConn2
  Transform Sensor1/RConn5 -- PS-Simulink Converter26/LConn1
  J1/RConn2 -- PS-Simulink Converter7/LConn1
  J4/RConn3 -- PS-Simulink Converter10/LConn1
  J6/RConn3 -- PS-Simulink Converter1/LConn1
  J5/RConn2 -- PS-Simulink Converter3/LConn1
  Simulink-PS Converter4/RConn1 -- J5/LConn2
  J3/RConn3 -- PS-Simulink Converter11/LConn1
  J7/RConn2 -- PS-Simulink Converter2/LConn1
  c3l3/LConn1 -- J3/RConn1
  Inertial Frame to EE/RConn4 -- PS-Simulink Converter16/LConn1
  Inertial Frame to EE/RConn6 -- PS-Simulink Converter18/LConn1
  J2/RConn2 -- PS-Simulink Converter6/LConn1
  c3l1/RConn1 -- J2/LConn1
  J7/RConn3 -- PS-Simulink Converter8/LConn1
  Simulink-PS Converter6/RConn1 -- J7/LConn2
  c3l1/LConn1 -- J1/RConn1
  Arm base to EE/RConn6 -- PS-Simulink Converter32/LConn1
  Arm base to EE/RConn10 -- PS-Simulink Converter36/LConn1
  PS-Simulink Converter34/LConn1 -- Arm base to EE/RConn8
  Arm base to EE/RConn9 -- PS-Simulink Converter35/LConn1
  Arm base to EE/RConn7 -- PS-Simulink Converter33/LConn1
  Arm base to EE/RConn11 -- PS-Simulink Converter37/LConn1
  PS-Simulink Converter31/LConn1 -- Arm base to EE/RConn5
  PS-Simulink Converter29/LConn1 -- Arm base to EE/RConn3
  Arm base to EE/RConn4 -- PS-Simulink Converter30/LConn1
  PS-Simulink Converter28/LConn1 -- Arm base to EE/RConn2
  Rigid Transform1/RConn1 -- Arm base to EE/LConn1
  Port1/RConn1 -- Port1rot1/LConn1
  Transform Sensor/RConn1 -- Cylindrical Solid/RConn1 -- Port1rot1/RConn1 -- Docking port/RConn1
  Transform Sensor/RConn3 -- PS-Simulink Converter38/LConn1
  PS-Simulink Converter39/LConn1 -- Transform Sensor/RConn4
  world/RConn1 -- 6-DOF Joint/LConn1
  PS-Simulink Converter42/LConn1 -- Transform Sensor2/RConn2
  Transform Sensor/LConn1 -- Port1/LConn1 -- Docked1/LConn1 -- 6-DOF Joint/RConn1 -- Concept3/LConn1 -- Transform Sensor1/RConn1 -- Transform Sensor2/LConn1
  Transform Sensor/RConn2 -- PS-Simulink Converter47/LConn1
  Inertial Frame to EE/RConn12 -- PS-Simulink Converter43/LConn1
  Transform Sensor1/RConn3 -- PS-Simulink Converter41/LConn1
  Transform Sensor1/RConn7 -- PS-Simulink Converter40/LConn1

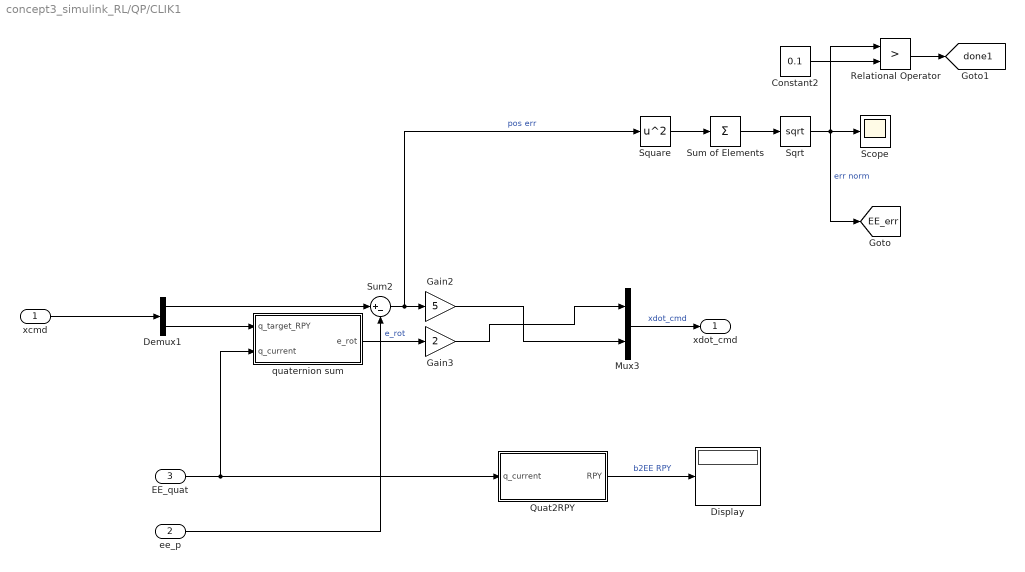
== system concept3_simulink_RL/QP/CLIK1 ==
  xcmd : Inport
  ee_p : Inport  Port=2
  EE_quat : Inport  Port=3
  Constant2 : Constant  Value=0.1
  Demux1 : Demux  Outputs=[3,3]
  Display : Display
  Gain2 : Gain  Gain=5
  Gain3 : Gain  Gain=2
  Mux3 : Mux  Inputs=2
  Quat2RPY : MATLAB Function  TreatAsAtomicUnit=on
  Relational Operator : RelationalOperator  Operator=>  OutDataTypeStr=boolean  RndMeth=Simplest  InputSameDT=off
  Scope : Scope
      settings: DataLoggingVariableName=ScopeData5
  Sqrt : Sqrt
  Square : Math  Operator=square
  Sum of Elements : Sum  Inputs=+
  Sum2 : Sum  Inputs=|+-
  quaternion sum : MATLAB Function  TreatAsAtomicUnit=on
  xdot_cmd : Outport
  tag scope: EE_err=global, done1=global
  wires:
  Demux1/1 -> Sum2/1
  Demux1/2 -> quaternion sum/1(q_target_RPY)
  quaternion sum/1(e_rot) -> Gain3/1  "e_rot"
  EE_quat/1 -> Quat2RPY/1(q_current), quaternion sum/2(q_current)
  ee_p/1 -> Sum2/2
  xcmd/1 -> Demux1/1
  Mux3/1 -> xdot_cmd/1  "xdot_cmd"
  Gain3/1 -> Mux3/1
  Gain2/1 -> Mux3/2
  Sum2/1 -> Square/1, Gain2/1  "pos err"
  Sum of Elements/1 -> Sqrt/1
  Square/1 -> Sum of Elements/1
  Sqrt/1 -> Relational Operator/1, [EE_err], Scope/1  "err norm"
  Constant2/1 -> Relational Operator/2
  Relational Operator/1 -> [done1]
  Quat2RPY/1(RPY) -> Display/1  "b2EE RPY"

== system concept3_simulink_RL/QP/Path-Planning  ==
  docked : Inport
  Clock : Clock
  MATLAB Function : MATLAB Function  TreatAsAtomicUnit=on
  MATLAB Function1 : MATLAB Function  TreatAsAtomicUnit=on
  MATLAB Function2 : MATLAB Function  Commented=on  TreatAsAtomicUnit=on
  MATLAB Function3 : MATLAB Function  Commented=on  TreatAsAtomicUnit=on
  MATLAB Function4 : MATLAB Function  TreatAsAtomicUnit=on
  Switch1 : Switch  Criteria=u2 > Threshold  SaturateOnIntegerOverflow=off  InputSameDT=off
  Switch2 : Switch  Criteria=u2 > Threshold  SaturateOnIntegerOverflow=off  InputSameDT=off
  To Workspace : ToWorkspace  VariableName=xdot_des  SaveFormat=Timeseries  SampleTime=-1
  ydot : Outport
  poly_traj_ab : Outport  Port=2
  wires:
  Clock/1 -> MATLAB Function1/1(clock), MATLAB Function4/1(clock)
  MATLAB Function/1(EE_pos) -> poly_traj_ab/1  "poly_traj_ab"
  docked/1 -> MATLAB Function1/2(docked), Switch1/2, Switch2/2, MATLAB Function/2(docked)
  Switch1/1 -> MATLAB Function/1(pos_rpy)
  MATLAB Function4/2(y) -> Switch1/3
  MATLAB Function4/1(ydot) -> Switch2/3
  Switch2/1 -> To Workspace/1, ydot/1
  MATLAB Function1/1(ydot) -> Switch2/1
  MATLAB Function1/2(y) -> Switch1/1

== system concept3_simulink_RL/QP/Subsystem1 ==
  xcmd : Inport
  ee_p : Inport  Port=2
  EE_quat : Inport  Port=3
  CLIK_fn : MATLAB Function  TreatAsAtomicUnit=on
  Display : Display
  Mux : Mux  Inputs=2
  Quat2RPY : MATLAB Function  TreatAsAtomicUnit=on
  To Workspace : ToWorkspace  VariableName=b2EE  SaveFormat=Timeseries  SampleTime=Tlog
  To Workspace1 : ToWorkspace  VariableName=x_cmd  SaveFormat=Timeseries  SampleTime=Tlog
  xdot_cmd : Outport
  tag scope: eee=global
  wires:
  EE_quat/1 -> Quat2RPY/1(q_current), CLIK_fn/3(EE_quat)
  xcmd/1 -> To Workspace1/1, CLIK_fn/1(xcmd)
  ee_p/1 -> Mux/1, CLIK_fn/2(ee_p)
  Quat2RPY/1(RPY) -> Mux/2, Display/1  "b2EE RPY"
  CLIK_fn/1(xdot_cmd) -> xdot_cmd/1
  CLIK_fn/2(pos_err) -> [eee]  "eee"
  Mux/1 -> To Workspace/1

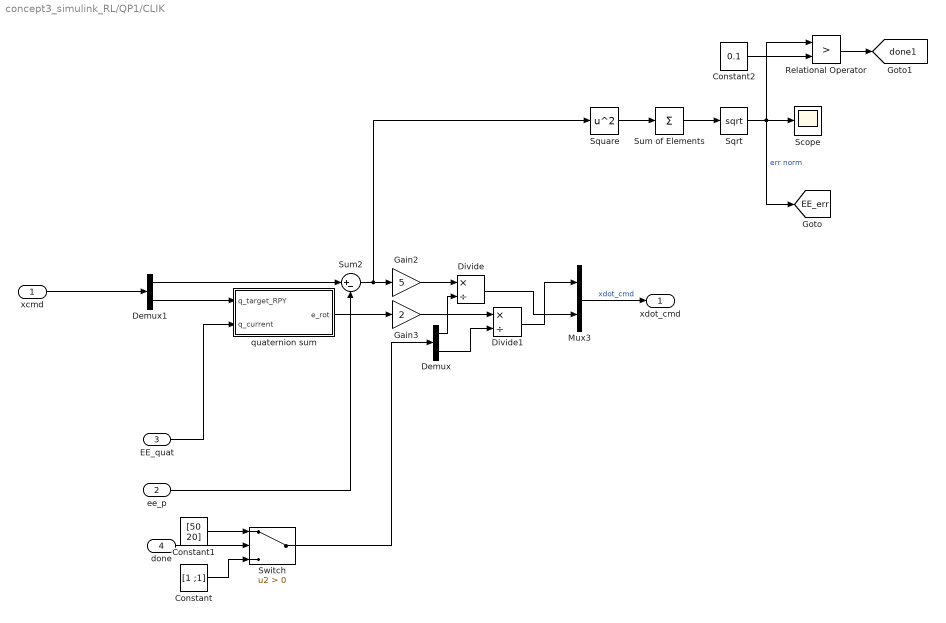
== system concept3_simulink_RL/QP1/CLIK ==
  xcmd : Inport
  ee_p : Inport  Port=2
  EE_quat : Inport  Port=3
  done : Inport  Port=4
  Constant : Constant  Value=[1 ;1]
  Constant1 : Constant  Value=[50 20]
  Constant2 : Constant  Value=0.1
  Demux : Demux  Outputs=2
  Demux1 : Demux  Outputs=[3,3]
  Divide : Product  Inputs=*/
  Divide1 : Product  Inputs=*/
  Gain2 : Gain  Gain=5
  Gain3 : Gain  Gain=2
  Mux3 : Mux  Inputs=2
  Relational Operator : RelationalOperator  Operator=>  OutDataTypeStr=boolean  RndMeth=Simplest  InputSameDT=off
  Scope : Scope
      settings: DataLoggingVariableName=ScopeData5
  Sqrt : Sqrt
  Square : Math  Operator=square
  Sum of Elements : Sum  Inputs=+
  Sum2 : Sum  Inputs=|+-
  Switch : Switch  Criteria=u2 > Threshold  SaturateOnIntegerOverflow=off  InputSameDT=off
  quaternion sum : MATLAB Function  TreatAsAtomicUnit=on
  xdot_cmd : Outport
  tag scope: EE_err=global, done1=global
  wires:
  Relational Operator/1 -> [done1]
  Constant2/1 -> Relational Operator/2
  Sqrt/1 -> Scope/1, [EE_err], Relational Operator/1  "err norm"
  Square/1 -> Sum of Elements/1
  Sum of Elements/1 -> Sqrt/1
  Sum2/1 -> Gain2/1, Square/1
  Switch/1 -> Demux/1
  Divide/1 -> Mux3/2
  Divide1/1 -> Mux3/1
  Demux/2 -> Divide1/2
  Demux/1 -> Divide/2
  done/1 -> Switch/2
  Constant1/1 -> Switch/1
  Constant/1 -> Switch/3
  Gain2/1 -> Divide/1
  Gain3/1 -> Divide1/1
  Mux3/1 -> xdot_cmd/1  "xdot_cmd"
  xcmd/1 -> Demux1/1
  ee_p/1 -> Sum2/2
  EE_quat/1 -> quaternion sum/2(q_current)
  quaternion sum/1(e_rot) -> Gain3/1
  Demux1/2 -> quaternion sum/1(q_target_RPY)
  Demux1/1 -> Sum2/1

== system concept3_simulink_RL/QP1/Subsystem ==
  In1 : Inport
  QP : MATLABFcn  MATLABFcn=QP_c3_RL  OutputDimensions=14
  qdot_cmd : Outport
  wires:
  QP/1 -> qdot_cmd/1  "qdot_cmd"
  In1/1 -> QP/1

== system concept3_simulink_RL/RL/stop ==
  In2 : Inport
  Constant1 : Constant  Value=0.5
  Relational Operator1 : RelationalOperator  OutDataTypeStr=boolean  RndMeth=Simplest  InputSameDT=off
  Selector1 : Selector  InputPortWidth=3  IndexOptions=Index vector (dialog)  Indices=[1 2]  OutputSizes=1
  Sqrt : Sqrt
  Square : Math  Operator=square
  Sum of Elements : Sum  Inputs=+
  Out1 : Outport
  wires:
  Relational Operator1/1 -> Out1/1
  In2/1 -> Selector1/1
  Selector1/1 -> Square/1
  Sum of Elements/1 -> Sqrt/1
  Square/1 -> Sum of Elements/1
  Sqrt/1 -> Relational Operator1/1
  Constant1/1 -> Relational Operator1/2

== system concept3_simulink_RL/Plant/Attach_logic/Attach sensor ==
  Atttach flip-flop : simulink_extras/Flip Flops/S-R Flip-Flop  initial_condition=0
  EE 2 target : sm_lib/Frames and Transforms/Transform Sensor  MeasurementFrame=World  RotationSequence=XYX  SenseAngle=off  SenseAxis=off  SenseQ=on  SenseR=off  SenseRotationSequence=off  SenseOmegaX=off  SenseOmegaY=off  SenseOmegaZ=off  SenseOmega=on  SenseQDot=off  SenseRDot=off  SenseRotationSequenceDot=off  SenseAlphaX=off  SenseAlphaY=off  SenseAlphaZ=off  SenseAlpha=off  SenseQDDot=off  SenseRDDot=off  SenseX=off  SenseY=off  SenseZ=off  SenseXYZ=on  SenseRad=off  SenseAzim=off  SenseDist=off  SenseInc=off  SenseXDot=off  SenseYDot=off  SenseZDot=off  SenseXYZDot=on  SenseRadDot=off  SenseAzimDot=off  SenseDistDot=off  SenseIncDot=off  SenseXDDot=off  SenseYDDot=off  SenseZDDot=off  SenseXYZDDot=off  SenseRadDDot=off  SenseAzimDDot=off  SenseDistDDot=off  SenseIncDDot=off
  NOT : Logic  Operator=NOT  IconShape=distinctive  AllPortsSameDT=off  OutDataTypeStr=boolean
  PS-Simulink Converter{2..5} (4 alike) : nesl_utility/PS-Simulink Converter  PhysicalDomain=network_engine_domain  SubClassName=ps_output  LeftPortType=input  RightPortType=output  PseudoPeriodic=off  Frequencies=[]  VectorFormat=inherit  Unit=inherit  AffineConversion=off
  S-R Flip-Flop : simulink_extras/Flip Flops/S-R Flip-Flop  initial_condition=0
  Subsystem : Subsystem
  Unit Delay : UnitDelay  SampleTime=-1  HasFrameUpgradeWarning=on
  EE : PMIOPort  Side=Left
  Sat : PMIOPort  Port=2  Side=Right
  attach : Outport
  wires:
  [docked] -> Atttach flip-flop/2
  Atttach flip-flop/1 -> S-R Flip-Flop/1, attach/1
  PS-Simulink Converter2/1 -> Subsystem/1(q_current)
  PS-Simulink Converter4/1 -> Subsystem/2(w)
  PS-Simulink Converter3/1 -> Subsystem/3(p)
  PS-Simulink Converter5/1 -> Subsystem/4(v)
  Subsystem/1(True attach) -> Atttach flip-flop/1
  NOT/1 -> Subsystem/Enable
  Unit Delay/1 -> NOT/1
  S-R Flip-Flop/1 -> Unit Delay/1
  connections:
  PS-Simulink Converter4/LConn1 -- EE 2 target/RConn3
  PS-Simulink Converter5/LConn1 -- EE 2 target/RConn5
  EE 2 target/RConn2 -- PS-Simulink Converter2/LConn1
  PS-Simulink Converter3/LConn1 -- EE 2 target/RConn4
  EE/RConn1 -- EE 2 target/LConn1
  EE 2 target/RConn1 -- Sat/RConn1

== system concept3_simulink_RL/Plant/Docking logic/Docking sensor ==
  Dock flip-flop : simulink_extras/Flip Flops/S-R Flip-Flop  initial_condition=0
  NOT : Logic  Operator=NOT  IconShape=distinctive  AllPortsSameDT=off  OutDataTypeStr=boolean
  PS-Simulink Converter{2..5} (4 alike) : nesl_utility/PS-Simulink Converter  PhysicalDomain=network_engine_domain  SubClassName=ps_output  LeftPortType=input  RightPortType=output  PseudoPeriodic=off  Frequencies=[]  VectorFormat=inherit  Unit=inherit  AffineConversion=off
  Subsystem : Subsystem
  Unit Delay : UnitDelay  SampleTime=-1  HasFrameUpgradeWarning=on
  port1 2 target : sm_lib/Frames and Transforms/Transform Sensor  MeasurementFrame=World  RotationSequence=XYX  SenseAngle=off  SenseAxis=off  SenseQ=on  SenseR=off  SenseRotationSequence=off  SenseOmegaX=off  SenseOmegaY=off  SenseOmegaZ=off  SenseOmega=on  SenseQDot=off  SenseRDot=off  SenseRotationSequenceDot=off  SenseAlphaX=off  SenseAlphaY=off  SenseAlphaZ=off  SenseAlpha=off  SenseQDDot=off  SenseRDDot=off  SenseX=off  SenseY=off  SenseZ=off  SenseXYZ=on  SenseRad=off  SenseAzim=off  SenseDist=off  SenseInc=off  SenseXDot=off  SenseYDot=off  SenseZDot=off  SenseXYZDot=on  SenseRadDot=off  SenseAzimDot=off  SenseDistDot=off  SenseIncDot=off  SenseXDDot=off  SenseYDDot=off  SenseZDDot=off  SenseXYZDDot=off  SenseRadDDot=off  SenseAzimDDot=off  SenseDistDDot=off  SenseIncDDot=off
  EE : PMIOPort  Side=Left
  Sat : PMIOPort  Port=2  Side=Right
  Dock : Outport
  wires:
  Dock flip-flop/1 -> Unit Delay/1, Dock/1
  PS-Simulink Converter2/1 -> Subsystem/1(q_current)
  PS-Simulink Converter4/1 -> Subsystem/2(w)
  PS-Simulink Converter3/1 -> Subsystem/3(p)
  PS-Simulink Converter5/1 -> Subsystem/4(v)
  Subsystem/1(True docking) -> Dock flip-flop/1
  NOT/1 -> Subsystem/Enable
  Unit Delay/1 -> NOT/1
  connections:
  PS-Simulink Converter4/LConn1 -- port1 2 target/RConn3
  PS-Simulink Converter5/LConn1 -- port1 2 target/RConn5
  port1 2 target/RConn2 -- PS-Simulink Converter2/LConn1
  PS-Simulink Converter3/LConn1 -- port1 2 target/RConn4
  EE/RConn1 -- port1 2 target/LConn1
  port1 2 target/RConn1 -- Sat/RConn1

== system concept3_simulink_RL/Plant/station_robot_arm/Concept3 ==
  Concept3_1_AxisTransform : sm_lib/Frames and Transforms/Rigid Transform  RotationMethod=ArbitraryAxis  FollAlignAxisA=+X  BaseAlignAxisA=+Y  FollAlignAxisB=+Y  BaseAlignAxisB=+Z  RotationStandardAxis=+Z  RotationAngle=0  RotationAngleUnits=rad  RotationArbitraryAxis=[1, 0, 0]  RotationSequenceAxes=FollowerAxes  RotationSequence=XYX  RotationSequenceAngles=[0 0 0]  RotationSequenceAnglesUnits=deg  RotationMatrix=[1 0 0;0 1 0;0 0 1]  Quaternion=[1 0 0 0]  TranslationMethod=Cartesian  TranslationCartesianOffset=[0, 0, 0]  TranslationCartesianOffsetUnits=m  TranslationStandardAxis=+Z  TranslationStandardOffset=0  TranslationStandardOffsetUnits=m  TranslationROffset=0  TranslationROffsetUnits=m  TranslationThetaOffset=0  TranslationThetaOffsetUnits=deg  TranslationZOffset=0  TranslationZOffsetUnits=m
  Concept3_1_OriginTransform : sm_lib/Frames and Transforms/Rigid Transform  RotationMethod=RotationSequence  FollAlignAxisA=+X  BaseAlignAxisA=+Y  FollAlignAxisB=+Y  BaseAlignAxisB=+Z  RotationStandardAxis=+Z  RotationAngle=0  RotationAngleUnits=deg  RotationArbitraryAxis=[0 0 1]  RotationSequenceAxes=BaseAxes  RotationSequence=XYZ  RotationSequenceAngles=[0, -0, 0]  RotationSequenceAnglesUnits=rad  RotationMatrix=[1 0 0;0 1 0;0 0 1]  Quaternion=[1 0 0 0]  TranslationMethod=Cartesian  TranslationCartesianOffset=[1.35, 0.225, 0.325]  TranslationCartesianOffsetUnits=m  TranslationStandardAxis=+Z  TranslationStandardOffset=0  TranslationStandardOffsetUnits=m  TranslationROffset=0  TranslationROffsetUnits=m  TranslationThetaOffset=0  TranslationThetaOffsetUnits=deg  TranslationZOffset=0  TranslationZOffsetUnits=m
  Concept3_visual : sm_lib/Body Elements/File Solid  ExtGeomFileName=meshes\Concept3.stl  UnitType=Custom  ExtGeomFileUnits=mm  StepReaderType=HEX  ExportConvexHullGeometry=off  InertiaType=Custom  BasedOnType=DensityFromFile  Density=1000  DensityUnits=kg/m^3  Mass=0  MassUnits=kg  CenterOfMass=[0, 0, 0]  CenterOfMassUnits=m  MomentsOfInertia=[0, 0, 0]  MomentsOfInertiaUnits=kg*m^2  ProductsOfInertia=[0, 0, 0]  ProductsOfInertiaUnits=kg*m^2  GraphicType=FromGeometry  MarkerShape=Sphere  MarkerSize=10  GraphicVisPropType=SimpleVisualProperties  GraphicDiffuseColor=[1 1 1]  GraphicOpacity=1  GraphicSpecularColor=[0.5 0.5 0.5 1.0]  GraphicAmbientColor=[0.15 0.15 0.15 1.0]  GraphicEmissiveColor=[0.0 0.0 0.0 1.0]  GraphicShininess=75  DoExposeReferenceFrame=on  SerializedFrames=<Frames/>
  Concept3_visualOriginTransform : sm_lib/Frames and Transforms/Rigid Transform  RotationMethod=RotationSequence  FollAlignAxisA=+X  BaseAlignAxisA=+Y  FollAlignAxisB=+Y  BaseAlignAxisB=+Z  RotationStandardAxis=+Z  RotationAngle=0  RotationAngleUnits=deg  RotationArbitraryAxis=[0 0 1]  RotationSequenceAxes=BaseAxes  RotationSequence=XYZ  RotationSequenceAngles=[0, 0, 0]  RotationSequenceAnglesUnits=rad  RotationMatrix=[1 0 0;0 1 0;0 0 1]  Quaternion=[1 0 0 0]  TranslationMethod=Cartesian  TranslationCartesianOffset=[0, 0, 0]  TranslationCartesianOffsetUnits=m  TranslationStandardAxis=+Z  TranslationStandardOffset=0  TranslationStandardOffsetUnits=m  TranslationROffset=0  TranslationROffsetUnits=m  TranslationThetaOffset=0  TranslationThetaOffsetUnits=deg  TranslationZOffset=0  TranslationZOffsetUnits=m
  Inertia1 : sm_lib/Body Elements/Inertia  InertiaType=Custom  Mass=3000  MassUnits=kg  CenterOfMass=[0, 0, 0]  CenterOfMassUnits=m  MomentsOfInertia=[776.884687974, 2512.766344178, 2739.139931228]  MomentsOfInertiaUnits=kg*m^2  ProductsOfInertia=[0.012030842, 0.07243477199999999, 0.050918524]  ProductsOfInertiaUnits=kg*m^2  GraphicType=None  MarkerShape=Inertia  MarkerSize=20  GraphicVisPropType=SimpleVisualProperties  GraphicDiffuseColor=[0.5 0.5 0.5]  GraphicOpacity=1  GraphicSpecularColor=[0.5 0.5 0.5 1.0]  GraphicAmbientColor=[0.15 0.15 0.15 1.0]  GraphicEmissiveColor=[0.0 0.0 0.0 1.0]  GraphicShininess=75
  InertiaOriginTransform : sm_lib/Frames and Transforms/Rigid Transform  RotationMethod=RotationSequence  FollAlignAxisA=+X  BaseAlignAxisA=+Y  FollAlignAxisB=+Y  BaseAlignAxisB=+Z  RotationStandardAxis=+Z  RotationAngle=0  RotationAngleUnits=deg  RotationArbitraryAxis=[0 0 1]  RotationSequenceAxes=BaseAxes  RotationSequence=XYZ  RotationSequenceAngles=[0, 0, 0]  RotationSequenceAnglesUnits=rad  RotationMatrix=[1 0 0;0 1 0;0 0 1]  Quaternion=[1 0 0 0]  TranslationMethod=Cartesian  TranslationCartesianOffset=[-0.005071042849789121, -1.252575805265672e-05, -1.78168660268183e-05]  TranslationCartesianOffsetUnits=m  TranslationStandardAxis=+Z  TranslationStandardOffset=0  TranslationStandardOffsetUnits=m  TranslationROffset=0  TranslationROffsetUnits=m  TranslationThetaOffset=0  TranslationThetaOffsetUnits=deg  TranslationZOffset=0  TranslationZOffsetUnits=m
  ReferenceFrame : sm_lib/Frames and Transforms/Reference Frame
  F : PMIOPort  Side=Left
  F1 : PMIOPort  Port=2  Side=Right
  connections:
  Concept3_1_AxisTransform/RConn1 -- F1/RConn1
  Concept3_1_AxisTransform/LConn1 -- Concept3_1_OriginTransform/RConn1
  Concept3_visual/RConn1 -- Concept3_visualOriginTransform/RConn1
  Inertia1/RConn1 -- InertiaOriginTransform/RConn1
  Concept3_visualOriginTransform/LConn1 -- InertiaOriginTransform/LConn1 -- Concept3_1_OriginTransform/LConn1 -- ReferenceFrame/RConn1 -- F/RConn1
